simulink model "AmModulation"  (R2015a)
settings: Solver=ode45  StartTime=0.0  StopTime=10.0  RelTol=1e-3
settings Model: Creator=Chayti  LastModifiedBy=hp

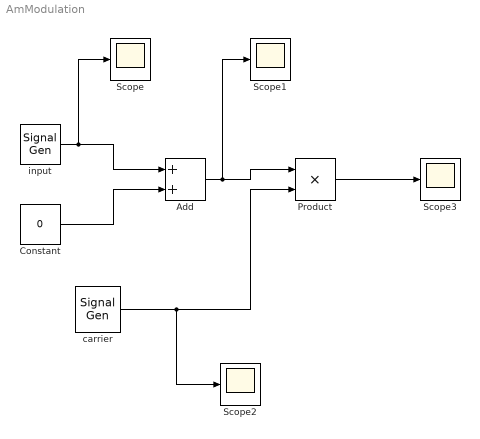
== system AmModulation ==
  Add : Sum
  Constant : Constant  Value=0
  Product : Product
  Scope{,1..3} (4 alike) : Scope
      Scope2 settings: SaveName=ScopeData2
      Scope3 settings: SaveName=ScopeData3
  carrier : SignalGenerator  Frequency=20
  input : SignalGenerator
  wires:
  input/1 -> Scope/1, Add/1
  Constant/1 -> Add/2
  Add/1 -> Scope1/1, Product/1
  carrier/1 -> Scope2/1, Product/2
  Product/1 -> Scope3/1
